simulink model "sim1"  (R2024b)
settings: Solver=VariableStepAuto  StartTime=0.0  StopTime=20  RelTol=1e-3
values from neighbouring files (symbols this model uses):
  c = 4    [sl1.m]
  d = 3    [sl1.m]
  j = 4    [sl1.m]
  T = 2    [sl1.m]
settings Model: Creator=cemal  LastModifiedBy=cemal

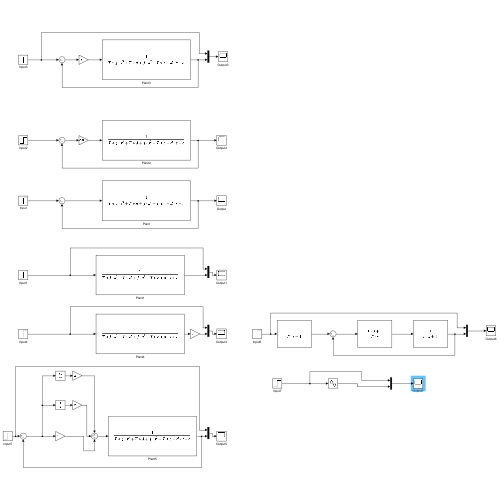
[thumbnail: Simulink's stored preview of the top-level diagram]
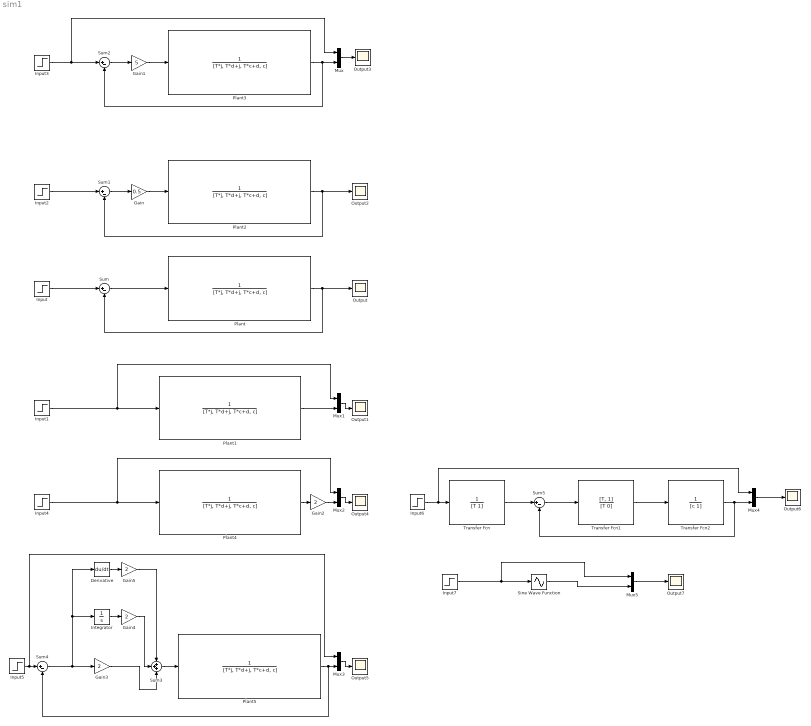
== system sim1 ==
  Derivative : Derivative
  Gain : Gain  Gain=0.5
  Gain1 : Gain  Gain=5
  Gain{2..5} (4 alike) : Gain  Gain=2
  Input{,1..7} (8 alike) : Step  SampleTime=0
  Integrator : Integrator
  Mux{,1..5} (6 alike) : Mux  Inputs=2
  Output{,1..7} (8 alike) : Scope
  Plant{,1..5} (6 alike) : TransferFcn  Denominator=[T*j, T*d+j, T*c+d, c]
  Sine Wave Function : Sin  TimeSource=Use external signal  SampleTime=0
  Sum{,1..2,4..5} (5 alike) : Sum  Inputs=|+-
  Sum3 : Sum  Inputs=+++
  Transfer Fcn : TransferFcn  Denominator=[T 1]
  Transfer Fcn1 : TransferFcn  Numerator=[T, 1]  Denominator=[T 0]
  Transfer Fcn2 : TransferFcn  Denominator=[c 1]
  wires:
  Input/1 -> Sum/1
  Plant/1 -> Sum/2, Output/1
  Sum/1 -> Plant/1
  Input1/1 -> Mux1/1, Plant1/1
  Plant1/1 -> Mux1/2
  Input2/1 -> Sum1/1
  Sum1/1 -> Gain/1
  Plant2/1 -> Sum1/2, Output2/1
  Gain/1 -> Plant2/1
  Sum2/1 -> Gain1/1
  Plant3/1 -> Mux/2, Sum2/2
  Input3/1 -> Mux/1, Sum2/1
  Gain1/1 -> Plant3/1
  Mux/1 -> Output3/1
  Mux1/1 -> Output1/1
  Plant4/1 -> Gain2/1
  Mux2/1 -> Output4/1
  Input4/1 -> Mux2/1, Plant4/1
  Gain2/1 -> Mux2/2
  Mux3/1 -> Output5/1
  Plant5/1 -> Sum4/2, Mux3/2
  Gain3/1 -> Sum3/3
  Integrator/1 -> Gain4/1
  Derivative/1 -> Gain5/1
  Sum3/1 -> Plant5/1
  Gain4/1 -> Sum3/2
  Gain5/1 -> Sum3/1
  Input5/1 -> Mux3/1, Sum4/1
  Sum4/1 -> Derivative/1, Integrator/1, Gain3/1
  Mux4/1 -> Output6/1
  Input6/1 -> Mux4/1, Transfer Fcn/1
  Transfer Fcn/1 -> Sum5/1
  Transfer Fcn2/1 -> Sum5/2, Mux4/2
  Transfer Fcn1/1 -> Transfer Fcn2/1
  Sum5/1 -> Transfer Fcn1/1
  Input7/1 -> Mux5/1, Sine Wave Function/1
  Mux5/1 -> Output7/1
  Sine Wave Function/1 -> Mux5/2
